simulink model "VFcontrol01"  (R2016a)
settings: Solver=FixedStepAuto  StartTime=0.0  StopTime=3  FixedStep=0.00005  RelTol=1e-3
values from neighbouring files (symbols this model uses):
  Lm = 0.1271    [motor4_workspace.mat]    (also in motor_wrapper.m = obj.Lm; scim_verifier.m = obj.motor.getLm(); setMotorParams.m; stationary_class.m = obj.Lm)
  Lr = 0.2744    [motor4_workspace.mat]    (also in motor_wrapper.m = obj.Lr; scim_verifier.m = obj.motor.getLr(); setMotorParams.m; stationary_class.m = obj.Lr)
  Ls = 0.2744    [motor4_workspace.mat]    (also in motor_wrapper.m = obj.Ls; scim_verifier.m = obj.motor.getLs(); setMotorParams.m; stationary.m = Ls/10)
  M_ab02abc = [1  0  1; -0.5  0.866025403784  1; -0.5  -0.866025403784  1]    [motor4_workspace.mat]    (also in setMotorParams.m = inv(M_abc2ab0); workspaceSav.mat)
  M_abc2ab0 = [0.666666666667  -0.333333333333  -0.333333333333; 0  0.57735026919  -0.57735026919; 0.333333333333  0.333333333333  0.333333333333]    [motor4_workspace.mat]    (also in setMotorParams.m = 2/3*[1, -0.5, -0.5; 0, sqrt(3)/2, -sqrt(3)/2;  0.5, 0.5, 0.5; workspaceSav.mat)
  p = 3    [getXYParam.m]    (also in plotXYParam.m; scim_verifier.m = real(is)*u; setMotorParams.m = 2)
  Rr = 1.009    [motor4_workspace.mat]    (also in motor_wrapper.m = obj.Rr; setMotorParams.m; stationary_class.m = obj.Rr; stationary_from_eq.m = obj.Rr)
  sig = (tox-fromx)/6    [gaussSpace.m]    (also in motor4_workspace.mat = 0.785452782217; setMotorParams.m = 0.785452782217; stationary_class.m = 1-Lm*Lm/Ls/Lr; torqueFinder.m = 0.785452782217)
libraries: simulink x1
settings Model: Creator=ebenera  LastModifiedBy=ebenera

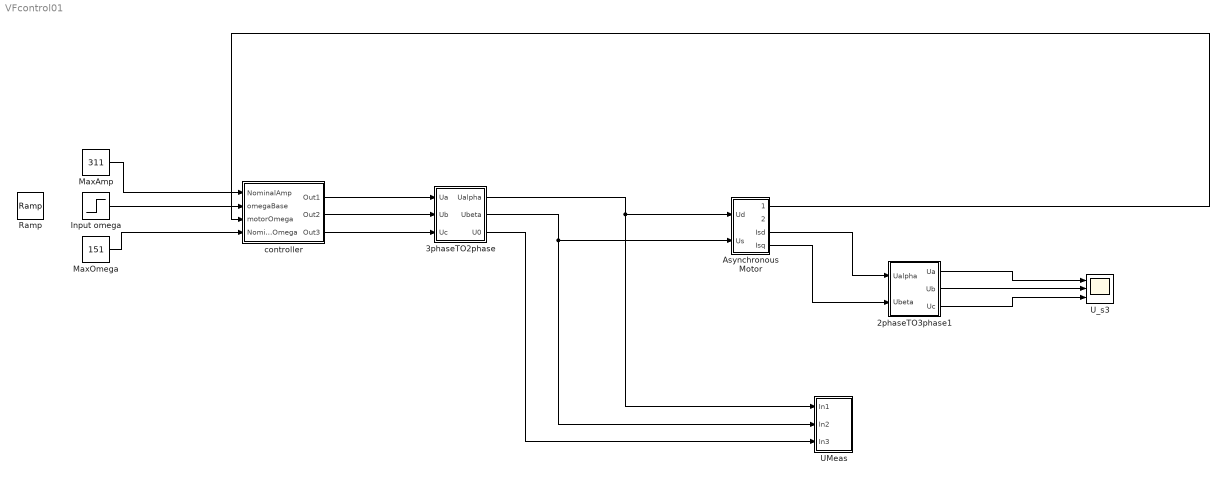
== system VFcontrol01 ==
  2phaseTO3phase1 : Subsystem
  "3phaseTO2phase " : Subsystem
  Asynchronous Motor : Subsystem
  Input omega : Step  Time=0.2  After=50  SampleTime=0
  MaxAmp : Constant  Value=311
  MaxOmega : Constant  Value=151
  Ramp : simulink/Sources/Ramp  slope=5  start=0  X0=1
  UMeas : Subsystem
  U_s3 : Scope  NumInputPorts=3
  controller : Subsystem
  wires:
  Asynchronous Motor/4(Isq) -> 2phaseTO3phase1/2(Ubeta)
  Asynchronous Motor/3(Isd) -> 2phaseTO3phase1/1(Ualpha)
  2phaseTO3phase1/1(Ua) -> U_s3/1
  2phaseTO3phase1/2(Ub) -> U_s3/2
  2phaseTO3phase1/3(Uc) -> U_s3/3
  MaxAmp/1 -> controller/1(NominalAmp)
  Input omega/1 -> controller/2(omegaBase)
  Asynchronous Motor/1(Omega) -> controller/3(motorOmega)
  MaxOmega/1 -> controller/4(NominalOmega)
  controller/1(Out1) -> "3phaseTO2phase "/1(Ua)
  controller/2(Out2) -> "3phaseTO2phase "/2(Ub)
  controller/3(Out3) -> "3phaseTO2phase "/3(Uc)
  "3phaseTO2phase "/1(Ualpha) -> Asynchronous Motor/1(Ud), UMeas/1(In1)
  "3phaseTO2phase "/2(Ubeta) -> Asynchronous Motor/2(Us), UMeas/2(In2)
  "3phaseTO2phase "/3(U0) -> UMeas/3(In3)

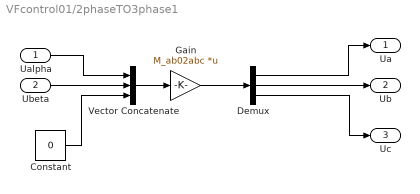
== system VFcontrol01/2phaseTO3phase1 ==
  Ualpha : Inport
  Ubeta : Inport  Port=2
  Constant : Constant  Value=0
  Demux : Demux  Outputs=3
  Gain : Gain  Gain=M_ab02abc  Multiplication=Matrix(K*u)
  Vector Concatenate : Concatenate  NumInputs=3
  Ua : Outport
  Ub : Outport  Port=2
  Uc : Outport  Port=3
  wires:
  Vector Concatenate/1 -> Gain/1
  Ualpha/1 -> Vector Concatenate/1
  Demux/3 -> Uc/1
  Gain/1 -> Demux/1
  Constant/1 -> Vector Concatenate/3
  Ubeta/1 -> Vector Concatenate/2
  Demux/1 -> Ua/1
  Demux/2 -> Ub/1

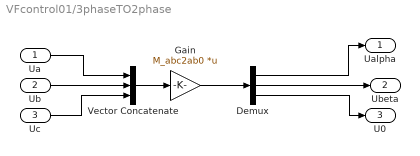
== system VFcontrol01/3phaseTO2phase  ==
  Ua : Inport
  Ub : Inport  Port=2
  Uc : Inport  Port=3
  Demux : Demux  Outputs=3
  Gain : Gain  Gain=M_abc2ab0  Multiplication=Matrix(K*u)
  Vector Concatenate : Concatenate  NumInputs=3
  Ualpha : Outport
  Ubeta : Outport  Port=2
  U0 : Outport  Port=3
  wires:
  Vector Concatenate/1 -> Gain/1
  Ua/1 -> Vector Concatenate/1
  Demux/3 -> U0/1
  Gain/1 -> Demux/1
  Uc/1 -> Vector Concatenate/3
  Ub/1 -> Vector Concatenate/2
  Demux/1 -> Ualpha/1
  Demux/2 -> Ubeta/1

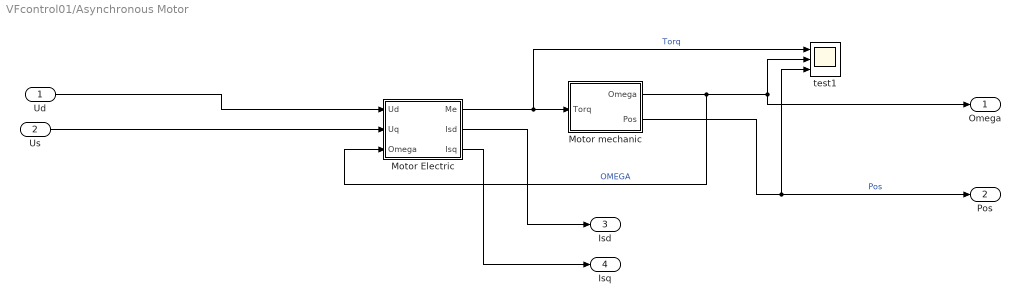
== system VFcontrol01/Asynchronous Motor ==
  Ud : Inport
  Us : Inport  Port=2
  Motor Electric : Subsystem
  Motor mechanic : Subsystem
  test1 : Scope  NumInputPorts=3
  Omega : Outport
  Pos : Outport  Port=2
  Isd : Outport  Port=3
  Isq : Outport  Port=4
  wires:
  Motor mechanic/2(Pos) -> test1/3, Pos/1  "Pos"
  Motor mechanic/1(Omega) -> test1/2, Omega/1, Motor Electric/3(Omega)  "OMEGA"
  Motor Electric/1(Me) -> test1/1, Motor mechanic/1("Torq ")  "Torq"
  Motor Electric/2(Isd) -> Isd/1
  Motor Electric/3(Isq) -> Isq/1
  Us/1 -> Motor Electric/2(Uq)
  Ud/1 -> Motor Electric/1(Ud)

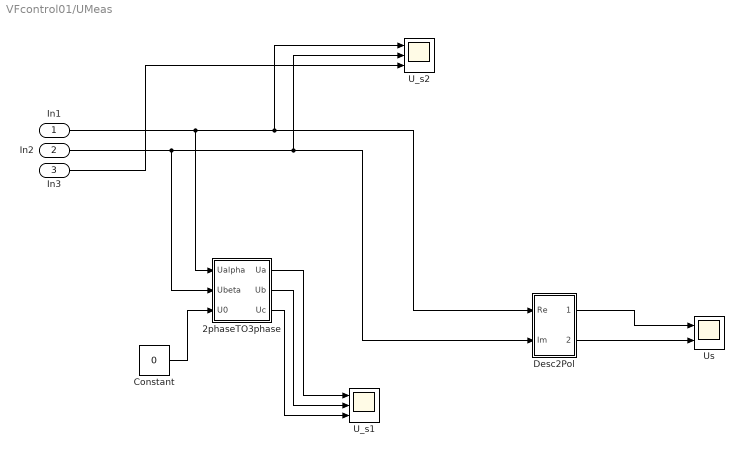
== system VFcontrol01/UMeas ==
  In1 : Inport
  In2 : Inport  Port=2
  In3 : Inport  Port=3
  2phaseTO3phase : Subsystem
  Constant : Constant  Value=0
  Desc2Pol : Subsystem
  U_s1 : Scope  NumInputPorts=3
  U_s2 : Scope  NumInputPorts=3
  Us : Scope  NumInputPorts=2
  wires:
  In1/1 -> 2phaseTO3phase/1(Ualpha), U_s2/1, Desc2Pol/1(Re)
  In2/1 -> 2phaseTO3phase/2(Ubeta), Desc2Pol/2(Im), U_s2/2
  Desc2Pol/1(Amp) -> Us/1
  Desc2Pol/2(Angle) -> Us/2
  In3/1 -> U_s2/3
  Constant/1 -> 2phaseTO3phase/3(U0)
  2phaseTO3phase/1(Ua) -> U_s1/1
  2phaseTO3phase/2(Ub) -> U_s1/2
  2phaseTO3phase/3(Uc) -> U_s1/3

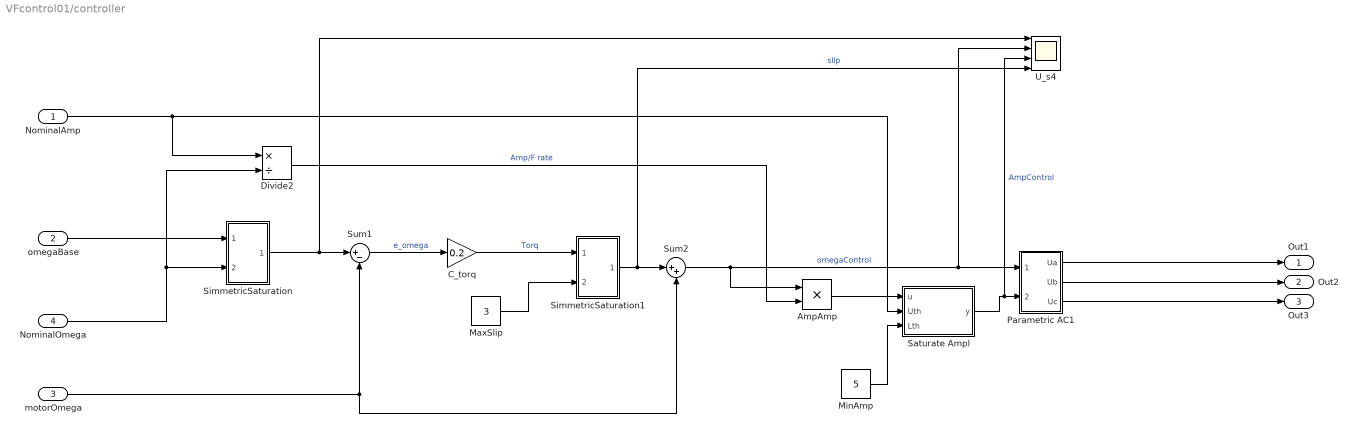
== system VFcontrol01/controller ==
  NominalAmp : Inport
  omegaBase : Inport  Port=2
  motorOmega : Inport  Port=3
  NominalOmega : Inport  Port=4
  AmpAmp : Product
  C_torq : Gain  Gain=0.2
  Divide2 : Product  Inputs=*/  SaturateOnIntegerOverflow=on  RndMeth=Zero
  MaxSlip : Constant  Value=3
  MinAmp : Constant  Value=5
  Parametric AC1 : Subsystem
  Saturate Ampl : MATLAB Function  TreatAsAtomicUnit=on
  SimmetricSaturation : Subsystem
  SimmetricSaturation1 : Subsystem
  Sum1 : Sum  Inputs=|+-
  Sum2 : Sum  Inputs=|++
  U_s4 : Scope  NumInputPorts=4
  Out1 : Outport
  Out2 : Outport  Port=2
  Out3 : Outport  Port=3
  wires:
  Parametric AC1/2(Ub) -> Out2/1
  Parametric AC1/1(Ua) -> Out1/1
  Parametric AC1/3(Uc) -> Out3/1
  motorOmega/1 -> Sum2/2, Sum1/2
  MaxSlip/1 -> SimmetricSaturation1/2(max)
  Sum1/1 -> C_torq/1  "e_omega"
  NominalAmp/1 -> Saturate Ampl/2(Uth), Divide2/1
  SimmetricSaturation1/1(Out1) -> U_s4/4, Sum2/1  "slip"
  MinAmp/1 -> Saturate Ampl/3(Lth)
  NominalOmega/1 -> Divide2/2, SimmetricSaturation/2(max)
  Saturate Ampl/1(y) -> U_s4/3, Parametric AC1/2(Amp)  "AmpControl"
  AmpAmp/1 -> Saturate Ampl/1(u)
  Sum2/1 -> AmpAmp/1, U_s4/2, Parametric AC1/1(Omega)  "omegaControl"
  Divide2/1 -> AmpAmp/2  "Amp/F rate"
  C_torq/1 -> SimmetricSaturation1/1(signal)  "Torq"
  SimmetricSaturation/1(Out1) -> U_s4/1, Sum1/1
  omegaBase/1 -> SimmetricSaturation/1(signal)

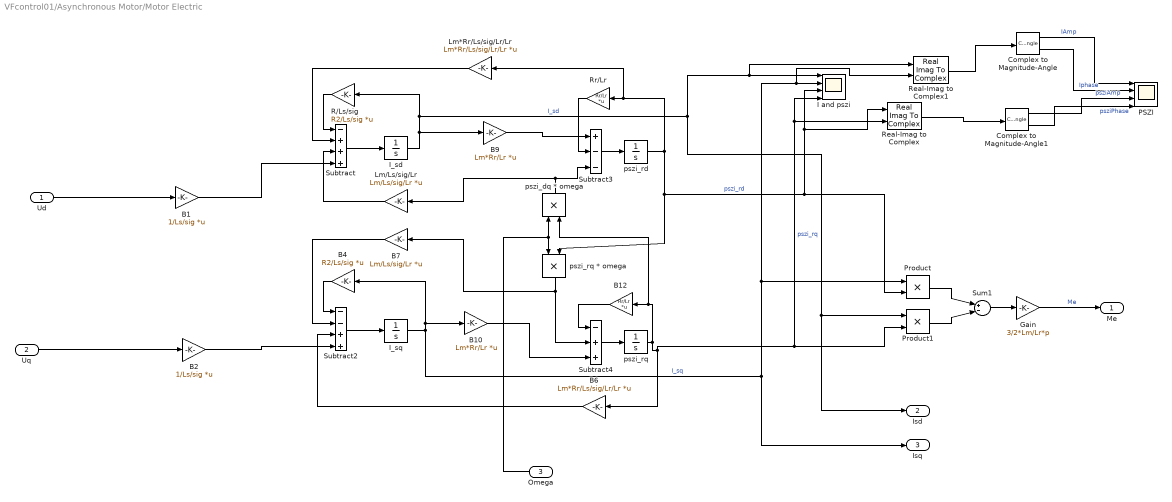
== system VFcontrol01/Asynchronous Motor/Motor Electric ==
  Ud : Inport
  Uq : Inport  Port=2
  Omega : Inport  Port=3
  B1 : Gain  Gain=1/Ls/sig  Multiplication=Matrix(K*u)
  B10 : Gain  Gain=Lm*Rr/Lr  Multiplication=Matrix(K*u)
  B12 : Gain  Gain=Rr/Lr  Multiplication=Matrix(K*u)
  B2 : Gain  Gain=1/Ls/sig  Multiplication=Matrix(K*u)
  B4 : Gain  Gain=R2/Ls/sig  Multiplication=Matrix(K*u)
  B6 : Gain  Gain=Lm*Rr/Ls/sig/Lr/Lr  Multiplication=Matrix(K*u)
  B7 : Gain  Gain=Lm/Ls/sig/Lr  Multiplication=Matrix(K*u)
  B9 : Gain  Gain=Lm*Rr/Lr  Multiplication=Matrix(K*u)
  Complex to Magnitude-Angle : ComplexToMagnitudeAngle
  Complex to Magnitude-Angle1 : ComplexToMagnitudeAngle
  Gain : Gain  Gain=3/2*Lm/Lr*p
  I and pszi : Scope  NumInputPorts=4
  I_sd : Integrator
  I_sq : Integrator
  Lm*Rr/Ls/sig/Lr/Lr : Gain  Gain=Lm*Rr/Ls/sig/Lr/Lr  Multiplication=Matrix(K*u)
  Lm/Ls/sig/Lr : Gain  Gain=Lm/Ls/sig/Lr  Multiplication=Matrix(K*u)
  PSZI : Scope  NumInputPorts=4
  Product : Product
  Product1 : Product
  R/Ls/sig : Gain  Gain=R2/Ls/sig  Multiplication=Matrix(K*u)
  Real-Imag to Complex : RealImagToComplex
  Real-Imag to Complex1 : RealImagToComplex
  Rr/Lr : Gain  Gain=Rr/Lr  Multiplication=Matrix(K*u)
  Subtract : Sum  Inputs=-+++
  Subtract2 : Sum  Inputs=--++
  Subtract3 : Sum  Inputs=+--
  Subtract4 : Sum  Inputs=-++
  Sum1 : Sum  Inputs=|+-|
  pszi_dq * omega : Product
  pszi_rd : Integrator
  "pszi_rq " : Integrator
  pszi_rq * omega : Product
  Me : Outport
  Isd : Outport  Port=2
  Isq : Outport  Port=3
  wires:
  pszi_rq * omega/1 -> Subtract4/2, B7/1
  Subtract/1 -> I_sd/1
  B12/1 -> Subtract4/1
  Product1/1 -> Sum1/2
  Lm*Rr/Ls/sig/Lr/Lr/1 -> Subtract/2
  Product/1 -> Sum1/1
  I_sq/1 -> Isq/1, Real-Imag to Complex1/2, I and pszi/2, Product/1, B10/1, B4/1  "I_sq"
  I_sd/1 -> B9/1, Isd/1, Product1/1, Real-Imag to Complex1/1, I and pszi/1, R/Ls/sig/1  "I_sd"
  Sum1/1 -> Gain/1
  R/Ls/sig/1 -> Subtract/1
  B6/1 -> Subtract2/3
  B4/1 -> Subtract2/1
  pszi_dq * omega/1 -> Subtract3/3, Lm/Ls/sig/Lr/1
  Omega/1 -> pszi_rq * omega/1, pszi_dq * omega/1
  B9/1 -> Subtract3/1
  Rr/Lr/1 -> Subtract3/2
  pszi_rd/1 -> Real-Imag to Complex/1, I and pszi/3, Product/2, pszi_rq * omega/2, Lm*Rr/Ls/sig/Lr/Lr/1, Rr/Lr/1  "pszi_rd"
  Lm/Ls/sig/Lr/1 -> Subtract/3
  "pszi_rq "/1 -> pszi_dq * omega/2, B12/1, Real-Imag to Complex/2, I and pszi/4, Product1/2, B6/1  "pszi_rq"
  B7/1 -> Subtract2/2
  Gain/1 -> Me/1  "Me"
  B10/1 -> Subtract4/3
  Subtract4/1 -> "pszi_rq "/1
  Subtract2/1 -> I_sq/1
  Subtract3/1 -> pszi_rd/1
  Uq/1 -> B2/1
  Ud/1 -> B1/1
  B1/1 -> Subtract/4
  B2/1 -> Subtract2/4
  Real-Imag to Complex1/1 -> Complex to Magnitude-Angle/1
  Complex to Magnitude-Angle/1 -> PSZI/1  "IAmp"
  Complex to Magnitude-Angle/2 -> PSZI/2  "Iphase"
  Real-Imag to Complex/1 -> Complex to Magnitude-Angle1/1
  Complex to Magnitude-Angle1/1 -> PSZI/3  "psziAmp"
  Complex to Magnitude-Angle1/2 -> PSZI/4  "psziPhase"

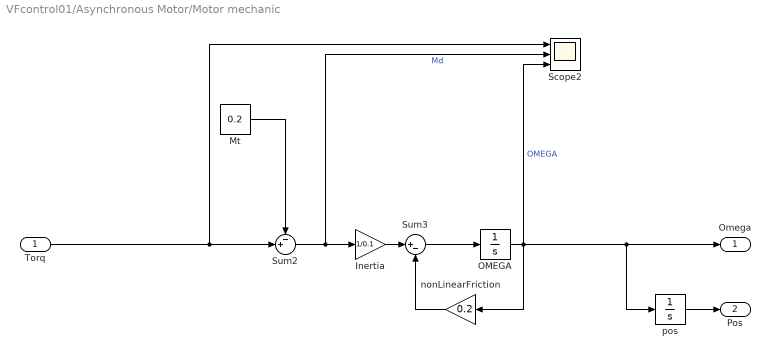
== system VFcontrol01/Asynchronous Motor/Motor mechanic ==
  "Torq " : Inport
  Inertia : Gain  Gain=1/0.1
  Mt : Constant  Value=0.2
  OMEGA : Integrator
  Scope2 : Scope  NumInputPorts=3
  Sum2 : Sum  Inputs=-+|
  Sum3 : Sum  Inputs=|+-
  nonLinearFriction : Gain  Gain=0.2
  pos : Integrator  WrapState=on
  Omega : Outport
  Pos : Outport  Port=2
  wires:
  "Torq "/1 -> Scope2/1, Sum2/2
  OMEGA/1 -> Scope2/3, pos/1, Omega/1, nonLinearFriction/1  "OMEGA"
  Sum3/1 -> OMEGA/1
  Sum2/1 -> Inertia/1, Scope2/2  "Md"
  Mt/1 -> Sum2/1
  nonLinearFriction/1 -> Sum3/2
  Inertia/1 -> Sum3/1
  pos/1 -> Pos/1

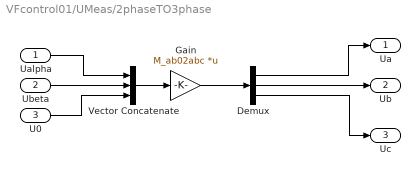
== system VFcontrol01/UMeas/2phaseTO3phase ==
  Ualpha : Inport
  Ubeta : Inport  Port=2
  U0 : Inport  Port=3
  Demux : Demux  Outputs=3
  Gain : Gain  Gain=M_ab02abc  Multiplication=Matrix(K*u)
  Vector Concatenate : Concatenate  NumInputs=3
  Ua : Outport
  Ub : Outport  Port=2
  Uc : Outport  Port=3
  wires:
  Vector Concatenate/1 -> Gain/1
  Ualpha/1 -> Vector Concatenate/1
  Demux/3 -> Uc/1
  Gain/1 -> Demux/1
  U0/1 -> Vector Concatenate/3
  Ubeta/1 -> Vector Concatenate/2
  Demux/1 -> Ua/1
  Demux/2 -> Ub/1

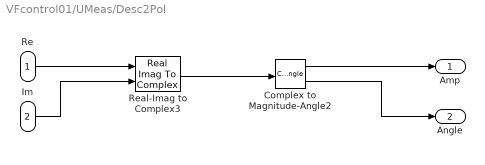
== system VFcontrol01/UMeas/Desc2Pol ==
  Re : Inport
  Im : Inport  Port=2
  Complex to Magnitude-Angle2 : ComplexToMagnitudeAngle
  Real-Imag to Complex3 : RealImagToComplex
  Amp : Outport
  Angle : Outport  Port=2
  wires:
  Complex to Magnitude-Angle2/1 -> Amp/1
  Real-Imag to Complex3/1 -> Complex to Magnitude-Angle2/1
  Complex to Magnitude-Angle2/2 -> Angle/1
  Re/1 -> Real-Imag to Complex3/1
  Im/1 -> Real-Imag to Complex3/2

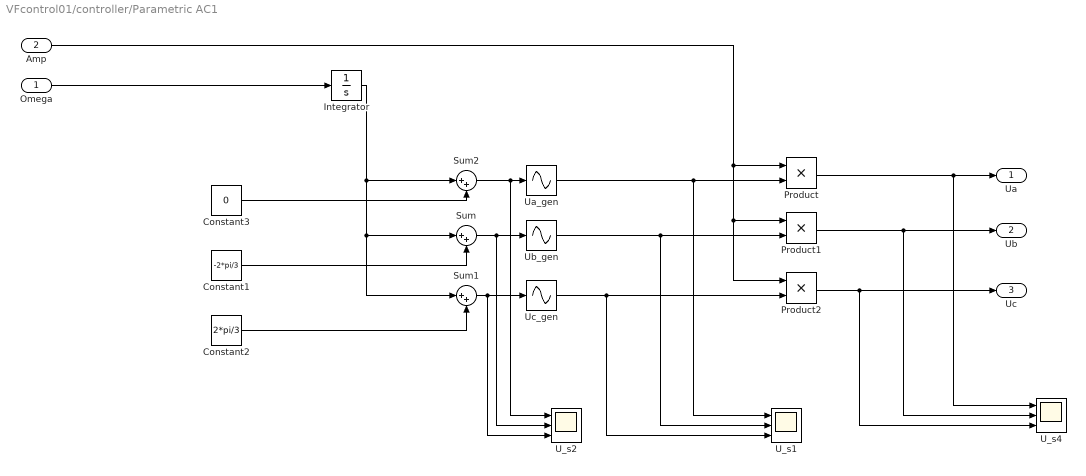
== system VFcontrol01/controller/Parametric AC1 ==
  Omega : Inport
  Amp : Inport  Port=2
  Constant1 : Constant  Value=-2*pi/3
  Constant2 : Constant  Value=2*pi/3
  Constant3 : Constant  Value=0
  Integrator : Integrator  WrapState=on
  Product : Product
  Product1 : Product
  Product2 : Product
  Sum : Sum  Inputs=|++
  Sum1 : Sum  Inputs=|++
  Sum2 : Sum  Inputs=|++
  U_s1 : Scope  NumInputPorts=3
  U_s2 : Scope  NumInputPorts=3
  U_s4 : Scope  NumInputPorts=3
  Ua_gen : Sin  TimeSource=Use external signal  SampleTime=0
  Ub_gen : Sin  TimeSource=Use external signal  SampleTime=0
  Uc_gen : Sin  TimeSource=Use external signal  SampleTime=0
  Ua : Outport
  Ub : Outport  Port=2
  Uc : Outport  Port=3
  wires:
  Sum/1 -> U_s2/2, Ub_gen/1
  Omega/1 -> Integrator/1
  Constant1/1 -> Sum/2
  Constant2/1 -> Sum1/2
  Sum1/1 -> U_s2/3, Uc_gen/1
  Sum2/1 -> U_s2/1, Ua_gen/1
  Constant3/1 -> Sum2/2
  Integrator/1 -> Sum2/1, Sum1/1, Sum/1
  Product/1 -> U_s4/1, Ua/1
  Product2/1 -> U_s4/3, Uc/1
  Product1/1 -> U_s4/2, Ub/1
  Amp/1 -> Product/1, Product1/1, Product2/1
  Ua_gen/1 -> U_s1/1, Product/2
  Uc_gen/1 -> U_s1/3, Product2/2
  Ub_gen/1 -> U_s1/2, Product1/2

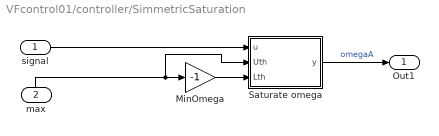
== system VFcontrol01/controller/SimmetricSaturation ==
  signal : Inport
  max : Inport  Port=2
  MinOmega : Gain  Gain=-1
  Saturate omega : MATLAB Function  TreatAsAtomicUnit=on
  Out1 : Outport
  wires:
  signal/1 -> Saturate omega/1(u)
  MinOmega/1 -> Saturate omega/3(Lth)
  Saturate omega/1(y) -> Out1/1  "omegaA"
  max/1 -> MinOmega/1, Saturate omega/2(Uth)

== system VFcontrol01/controller/SimmetricSaturation1 ==
  signal : Inport
  max : Inport  Port=2
  MinOmega : Gain  Gain=-1
  Saturate omega : MATLAB Function  TreatAsAtomicUnit=on
  Out1 : Outport
  wires:
  signal/1 -> Saturate omega/1(u)
  MinOmega/1 -> Saturate omega/3(Lth)
  Saturate omega/1(y) -> Out1/1  "omegaA"
  max/1 -> MinOmega/1, Saturate omega/2(Uth)

== matlab function VFcontrol01/controller/Saturate Ampl ==
  data: u input; y output; Uth input; Lth input
function y = fcn(u, Uth, Lth)
%#Uth is the UpperThreshold
% Lth is the LowerThreshold of the saturation
    y = min(u, Uth);
    y = max(y, Lth);
    
end

== matlab function VFcontrol01/controller/SimmetricSaturation/Saturate omega ==
  data: u input; y output; Uth input; Lth input
function y = fcn(u, Uth, Lth)
%#Uth is the UpperThreshold
% Lth is the LowerThreshold of the saturation
    y = min(u, Uth);
    y = max(y, Lth);
    
end

== matlab function VFcontrol01/controller/SimmetricSaturation1/Saturate omega ==
  data: u input; y output; Uth input; Lth input
function y = fcn(u, Uth, Lth)
%#Uth is the UpperThreshold
% Lth is the LowerThreshold of the saturation
    y = min(u, Uth);
    y = max(y, Lth);
    
end
